simulink model "K_LAZY"  (Simulink 7.7)
settings: Solver=ode3  StartTime=0.0  StopTime=10.0  FixedStep=5  RelTol=1e-3
settings Model: Creator=danwheeler  LastModifiedBy=danwheeler
settings DataIOCC: ExternalInput=UT  LoadExternalInput=on  SaveCompleteFinalSimState=on

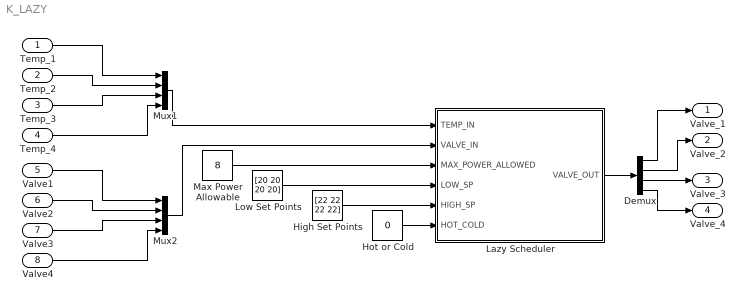
== system K_LAZY ==
  Temp_1 : Inport
  Temp_2 : Inport  Port=2
  Temp_3 : Inport  Port=3
  Temp_4 : Inport  Port=4
  Valve1 : Inport  Port=5
  Valve2 : Inport  Port=6
  Valve3 : Inport  Port=7
  Valve4 : Inport  Port=8
  Demux : Demux
  High Set Points : Constant  Value=[22 22 22 22]
  Hot or Cold : Constant  Value=0
  Lazy Scheduler : Stateflow chart  TreatAsAtomicUnit=on
  Low Set Points : Constant  Value=[20 20 20 20]
  Max Power Allowable : Constant  Value=8
  Mux1 : Mux
  Mux2 : Mux
  Valve_1 : Outport
  Valve_2 : Outport  Port=2
  Valve_3 : Outport  Port=3
  Valve_4 : Outport  Port=4
  wires:
  Temp_1/1 -> Mux1/1
  Temp_2/1 -> Mux1/2
  Temp_3/1 -> Mux1/3
  Temp_4/1 -> Mux1/4
  Mux1/1 -> Lazy Scheduler/1(TEMP_IN)
  Lazy Scheduler/1(VALVE_OUT) -> Demux/1
  Demux/1 -> Valve_1/1
  Demux/2 -> Valve_2/1
  Demux/3 -> Valve_3/1
  Demux/4 -> Valve_4/1
  Valve1/1 -> Mux2/1
  Valve2/1 -> Mux2/2
  Valve3/1 -> Mux2/3
  Valve4/1 -> Mux2/4
  Mux2/1 -> Lazy Scheduler/2(VALVE_IN)
  Max Power Allowable/1 -> Lazy Scheduler/3(MAX_POWER_ALLOWED)
  Low Set Points/1 -> Lazy Scheduler/4(LOW_SP)
  High Set Points/1 -> Lazy Scheduler/5(HIGH_SP)
  Hot or Cold/1 -> Lazy Scheduler/6(HOT_COLD)

== matlab function Lazy Scheduler ==
  data: TEMP_IN input double; VALVE_IN input double; MAX_POWER_ALLOWED input double; LOW_SP input double; HIGH_SP input double; VALVE_OUT output double; HOT_COLD input double
function VALVE_OUT = fcn(TEMP_IN,VALVE_IN,MAX_POWER_ALLOWED,LOW_SP,HIGH_SP,HOT_COLD)

CriticalStates = [0 0 0 0];
DesiredStates = [0 0 0 0];

basePower = 4.3;                                                           % Minimum power to run blower
powerPerAngle = 0.0186;                                                    % Power increase per servo angle
MAX_ALLOWED_ANGLES = ( MAX_POWER_ALLOWED - basePower ) / powerPerAngle;    % Total number of valve angles that are allowed

thresh = 0.1*(HIGH_SP-LOW_SP);                                             % Threshold values for critical states

%VALVE_OUT = VALVE_IN;                                                      % Initialize output variable
VALVE_OUT = [90 90 90 90];

% 
% COOLING
%
if HOT_COLD == 0
    %
    % TURN OFF ANY STATES THAT REACH LOW POINT
    %
    for i = 1:4
        if TEMP_IN(i) <= LOW_SP(i) %&& VALVE_IN(i) <= 90
            VALVE_OUT(i) = 90;
            VALVE_IN(i) = 90;   % Workaround for DETERMINE DESIRED STATES
        end 
    end

    %
    % FIND CRITICAL STATES, TURN THEM ALL ON
    %
    for i = 1:4
        if TEMP_IN(i) >= ( HIGH_SP(i)-thresh(i) )
            CriticalStates(i) = 1;
            VALVE_OUT(i) = 0;
        end    
    end
%
% HEATING
%
elseif HOT_COLD == 1
    %
    % TURN OFF ANY STATES THAT REACH HIGH POINT
    %
    for i = 1:4
        if TEMP_IN(i) >= HIGH_SP(i) %&& VALVE_IN(i) <= 90
            VALVE_OUT(i) = 90;
            VALVE_IN(i) = 90;   % Workaround for DETERMINE DESIRED STATES
        end 
    end

    %
    % FIND CRITICAL STATES, TURN THEM ALL ON
    %
    for i = 1:4
        if TEMP_IN(i) <= LOW_SP(i)                                         % Make critical when it falls below the low set point
            CriticalStates(i) = 1;
            VALVE_OUT(i) = 0;
        elseif TEMP_IN(i) <= ( LOW_SP(i) + thresh(i) ) && VALVE_IN(i) < 90 % Keep the state critical if it is on and within 10% of low threshold
            CriticalStates(i) = 1;
            VALVE_OUT(i) = 0;
        end    
    end
end

%
% DETERMINE DESIRED STATES
%
for i = 1:4
    if VALVE_IN(i) < 90                                                    % If the state was on, make it desired
        DesiredStates(i) = 1;
    end      
end
DesiredStates( CriticalStates == 1 ) = 0;

%CriticalStates
%DesiredStates

t = 360 - sum( VALVE_OUT );                                                % Total angle open of all valves
k = sum(CriticalStates);                                                   % Total number of critical states
m = sum(DesiredStates);                                                    % Total number of desired states

%
% HANDLE CRITICAL STATES
%
if k*90 > MAX_ALLOWED_ANGLES                                               % If you cant turn all the critical states completely on
    if k*50 > MAX_ALLOWED_ANGLES                                           % ... Make sure states are open at least 40 degrees
        VALVE_OUT( CriticalStates == 1 ) = 40;                             % ^
        VALVE_OUT( CriticalStates ~= 1 ) = 90;                             % ^ close the other states
        return
    else                                                                   % ... Open states as much as you can
        VALVE_OUT( CriticalStates == 1 ) = 90 - ( MAX_ALLOWED_ANGLES / k );
        VALVE_OUT( CriticalStates ~= 1 ) = 90;
        VALVE_OUT = floor( VALVE_OUT );
        VALVE_OUT( VALVE_OUT > 90 ) = 90;
        return
    end 
else                                                                       % Turn all the critical states completely on
    VALVE_OUT( CriticalStates == 1 ) = 0;
end

%
% HANDLE DESIRED STATES
%
MAX_ALLOWED_ANGLES = MAX_ALLOWED_ANGLES - ( sum( 90 - VALVE_OUT( CriticalStates == 1 ) ) ); % Determine remaining angles left
% Cooling
if HOT_COLD == 0
    mag = DesiredStates' .* ( TEMP_IN - LOW_SP );
% Heating
else
    mag = DesiredStates' .* ( HIGH_SP - TEMP_IN );
end
total = sum( mag );
temp = MAX_ALLOWED_ANGLES * ( mag / total );
VALVE_OUT( DesiredStates == 1 ) = 90 - temp( DesiredStates == 1 );
    
VALVE_OUT = floor( VALVE_OUT );
VALVE_OUT( VALVE_OUT > 90 ) = 90;
